simulink model "Sim4"  (R2021b)
settings: Solver=VariableStepAuto  StartTime=0.0  StopTime=90000  RelTol=1e-3
settings Model: Creator=Rasoul  LastModifiedBy=Rasoul
settings SolverCC: AlgebraicLoopSolver=TrustRegion
settings DebuggingCC: ArithmeticOperatorsInVariantConditions=warning
settings SFSimCC: CustomCodeUndefinedFunction=UseInterfaceOnly

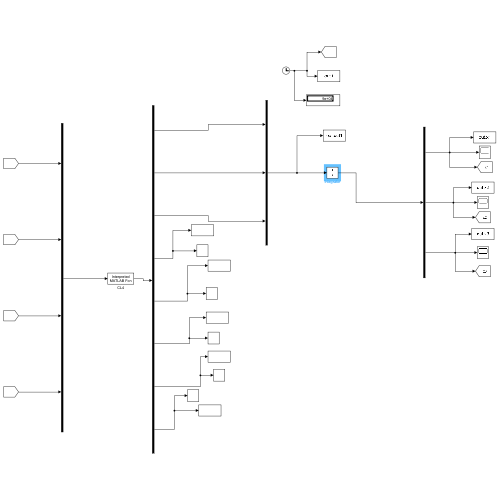
[thumbnail: Simulink's stored preview of the top-level diagram]
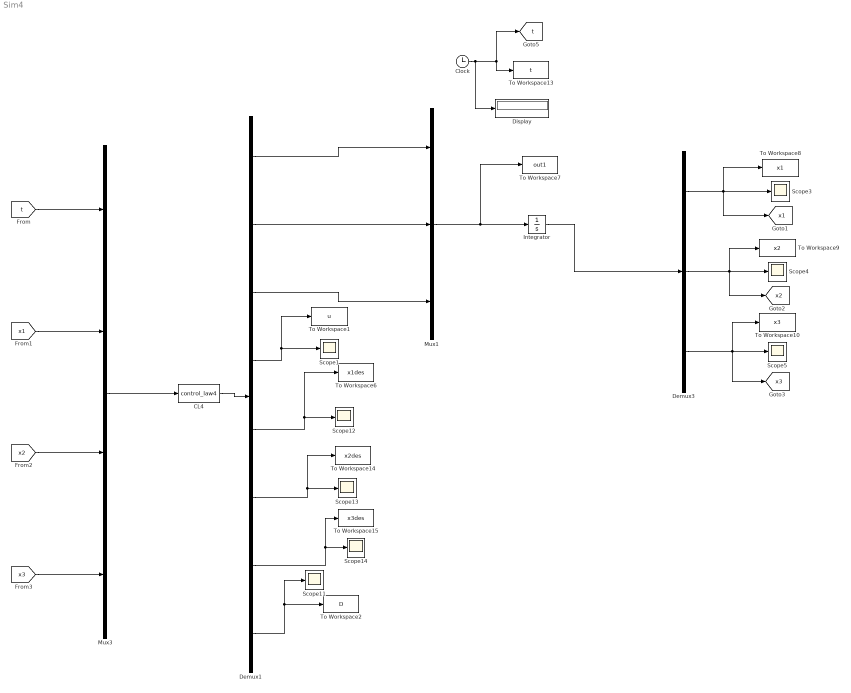
== system Sim4 ==
  CL4 : MATLABFcn  MATLABFcn=control_law4  OutputDimensions=8
  Clock : Clock
  Demux1 : Demux  Outputs=8
  Demux3 : Demux  Outputs=3
  Display : Display
  Integrator : Integrator  InitialCondition=[132;0;100]
  Mux1 : Mux  Inputs=3
  Mux3 : Mux
  Scope{1,3..5,11..14} (8 alike) : Scope
  To Workspace1 : ToWorkspace  VariableName=u  SampleTime=10
      settings: Save2DSignal=2-D array (concatenate along first dimension)
  To Workspace10 : ToWorkspace  VariableName=x3  SampleTime=10
      settings: Save2DSignal=2-D array (concatenate along first dimension)
  To Workspace13 : ToWorkspace  VariableName=t  SampleTime=10
      settings: Save2DSignal=2-D array (concatenate along first dimension)
  To Workspace14 : ToWorkspace  VariableName=x2des  SampleTime=10
      settings: Save2DSignal=2-D array (concatenate along first dimension)
  To Workspace15 : ToWorkspace  VariableName=x3des  SampleTime=10
      settings: Save2DSignal=2-D array (concatenate along first dimension)
  To Workspace2 : ToWorkspace  VariableName=D  SampleTime=10
      settings: Save2DSignal=2-D array (concatenate along first dimension)
  To Workspace6 : ToWorkspace  VariableName=x1des  SampleTime=10
      settings: Save2DSignal=2-D array (concatenate along first dimension)
  To Workspace7 : ToWorkspace  VariableName=out1  SampleTime=-1
      settings: Save2DSignal=2-D array (concatenate along first dimension)
  To Workspace8 : ToWorkspace  VariableName=x1  SampleTime=10
      settings: Save2DSignal=2-D array (concatenate along first dimension)
  To Workspace9 : ToWorkspace  VariableName=x2  SampleTime=10
      settings: Save2DSignal=2-D array (concatenate along first dimension)
  tag scope: t=global, x1=global, x2=global, x3=global
  wires:
  Mux1/1 -> To Workspace7/1, Integrator/1
  [x2] -> Mux3/3
  Demux3/1 -> [x1], Scope3/1, To Workspace8/1
  Demux3/3 -> [x3], Scope5/1, To Workspace10/1
  [x3] -> Mux3/4
  [x1] -> Mux3/2
  Mux3/1 -> CL4/1
  Demux1/1 -> Mux1/1
  Demux1/3 -> Mux1/3
  Clock/1 -> Display/1, [t], To Workspace13/1
  [t] -> Mux3/1
  Demux3/2 -> [x2], Scope4/1, To Workspace9/1
  Demux1/2 -> Mux1/2
  Demux1/5 -> To Workspace6/1, Scope12/1
  Demux1/6 -> To Workspace14/1, Scope13/1
  Demux1/7 -> To Workspace15/1, Scope14/1
  Integrator/1 -> Demux3/1
  CL4/1 -> Demux1/1
  Demux1/8 -> Scope11/1, To Workspace2/1
  Demux1/4 -> To Workspace1/1, Scope1/1
